simulink model "ECE_431_Homework_6"  (R2017a)
settings: Solver=FixedStepAuto  StartTime=0.0  StopTime=.1  FixedStep=1e-6  MaxStep=1e-4  RelTol=1e-3  EnableMultiTasking=on
undefined symbols (not defined in the file or in its folder): why
libraries: powerlib x9, powerlib_meascontrol x1
settings Model: Creator=Thomas  LastModifiedBy=Kenzie Brian

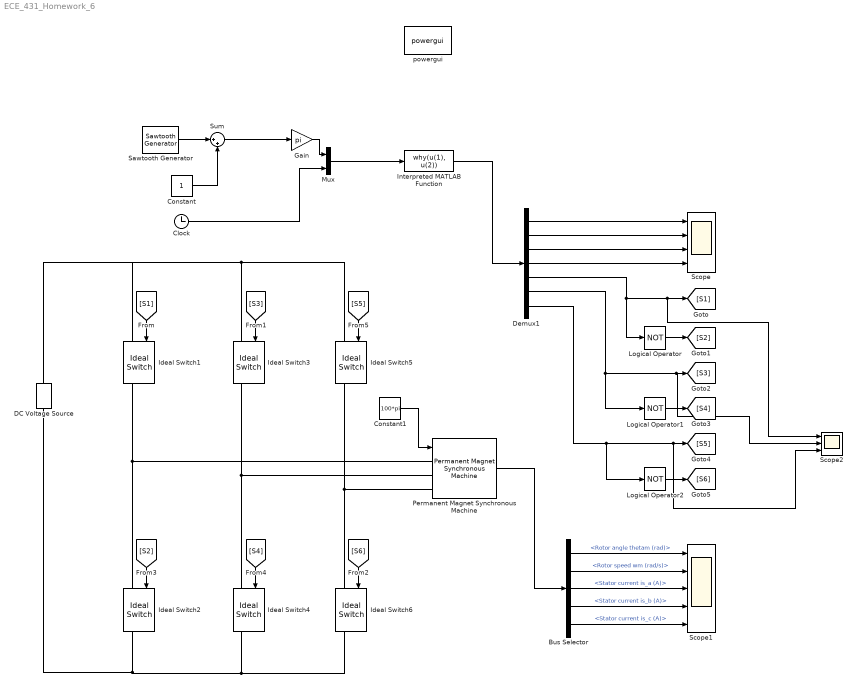
== system ECE_431_Homework_6 ==
  Bus Selector : BusSelector  OutputSignals=Rotor angle thetam (rad),Rotor speed wm (rad/s),Stator current is_a (A),Stator current is_b (A),Stator current is_c (A)
  Clock : Clock
      settings: Decimation=10000
  Constant : Constant
  Constant1 : Constant  Value=100*pi
  DC Voltage Source : powerlib/Electrical Sources/DC Voltage Source  Amplitude=280  Measurements=None
  Demux1 : Demux  Outputs=7
  Gain : Gain  Gain=pi
  Ideal Switch{1..6} (6 alike) : powerlib/Power Electronics/Ideal Switch  Ron=.01  Lon=0  IC=0  Rs=1e5  Cs=inf  Measurements=on
  Interpreted MATLAB Function : MATLABFcn  MATLABFcn=why(u(1), u(2))  Output1D=off
  Logical Operator : Logic  Operator=NOT  AllPortsSameDT=off  OutDataTypeStr=boolean
  Logical Operator1 : Logic  Operator=NOT  AllPortsSameDT=off  OutDataTypeStr=boolean
  Logical Operator2 : Logic  Operator=NOT  AllPortsSameDT=off  OutDataTypeStr=boolean
  Mux : Mux  Inputs=2
  Permanent Magnet Synchronous Machine : powerlib/Machines/Permanent Magnet Synchronous Machine  NbPhases=3  FluxDistribution=Sinusoidal  RotorType=Round  MechanicalLoad=Speed w  PresetModel=No  ShowDetailedParameters=on  MeasurementBus=off  Resistance=0.02  Inductance=8.5e-3  dqInductances=[8.5e-3,8.5e-3]  La=0.0002  MachineConstant=Flux linkage established by magnets (V.s)  Flux=0.03  VoltageCst=21.7656  TorqueCst=0.18  Flat=120  Mechanical=[0.1 0.003 8 0]  PolePairs=4  InitialConditions=[100*pi,0, 0,0]  InitialConditions5ph=[0 0 0 0 0 0]  TsPowergui=0  TsBlock=-1  RefAngle=90 degrees behind phase A axis (modified Park)
      settings: SourceProductName=Simscape Power Systems
  Sawtooth Generator : powerlib_meascontrol/Pulse & Signal Generators/Sawtooth Generator  Freq=100  Phase=180  Ts=0
      settings: SourceProductName=Simscape Power Systems
  Scope : Scope  NumInputPorts=4
  Scope1 : Scope  NumInputPorts=5
  Scope2 : Scope  NumInputPorts=3
  Sum : Sum  Inputs=|++
  powergui : powerlib/powergui  Priority=1  SimulationMode=Discrete  SampleTime=1e-6  frequency=60  Iterations=50  frequencyindice=0  Pbase=100e6  ErrMax=1e-4  UnitsV=kV  UnitsW=MW  buscounter=0  FunctionMessages=off  echomessages=off  EnableUseOfTLC=off  CurrentSourceSwitches=off  DisableSnubberDevices=off  DisableRonSwitches=off  DisableVfSwitches=off  DisplayEquations=off  SolverType=Tustin/Backward Euler (TBE)  Interpol=off  ExternalGateDelay=off  methode=off  Ts=100  x0status=blocks  SPID=off  SwTol=0  HookPort=off  RestoreLinks=warning  ResistiveCurrentMeasurement=off  Frange=[0:2:500]  Ylog=off  Xlog=on  ShowGrid=off  save=off  variable=ZData  structure=0  ZoomFFT=off  StartTime=0.0  cycles=1  DisplayStyle=1  fundamental=60  FreqAxis=off  MaxFrequency=1000  frequencyindicesteady=1  RmsSteady=1  display=off
  wires:
  Sawtooth Generator/1 -> Sum/1
  Mux/1 -> Interpreted MATLAB Function/1
  Constant/1 -> Sum/2
  Clock/1 -> Mux/2
  Demux1/2 -> Scope/2
  Demux1/3 -> Scope/3
  Sum/1 -> Gain/1
  Demux1/1 -> Scope/1
  Interpreted MATLAB Function/1 -> Demux1/1
  Demux1/4 -> Scope/4
  Gain/1 -> Mux/1
  [S3] -> Ideal Switch3/1
  [S1] -> Ideal Switch1/1
  [S5] -> Ideal Switch5/1
  [S2] -> Ideal Switch2/1
  [S4] -> Ideal Switch4/1
  [S6] -> Ideal Switch6/1
  Logical Operator/1 -> [S2]
  Logical Operator2/1 -> [S6]
  Logical Operator1/1 -> [S4]
  Demux1/6 -> Scope2/2, [S3], Logical Operator1/1
  Demux1/5 -> Scope2/1, [S1], Logical Operator/1
  Demux1/7 -> Scope2/3, [S5], Logical Operator2/1
  Permanent Magnet Synchronous Machine/1 -> Bus Selector/1
  Bus Selector/1 -> Scope1/1  "<Rotor angle thetam (rad)>"
  Bus Selector/2 -> Scope1/2  "<Rotor speed wm (rad/s)>"
  Bus Selector/3 -> Scope1/3  "<Stator current is_a (A)>"
  Bus Selector/4 -> Scope1/4  "<Stator current is_b (A)>"
  Bus Selector/5 -> Scope1/5  "<Stator current is_c (A)>"
  Constant1/1 -> Permanent Magnet Synchronous Machine/1
  connections:
  Ideal Switch2/LConn1 -- Permanent Magnet Synchronous Machine/LConn1 -- Ideal Switch1/RConn1
  Ideal Switch3/RConn1 -- Permanent Magnet Synchronous Machine/LConn2 -- Ideal Switch4/LConn1
  Ideal Switch6/LConn1 -- Permanent Magnet Synchronous Machine/LConn3 -- Ideal Switch5/RConn1
  Ideal Switch5/LConn1 -- DC Voltage Source/RConn1 -- Ideal Switch1/LConn1 -- Ideal Switch3/LConn1
  Ideal Switch2/RConn1 -- DC Voltage Source/LConn1 -- Ideal Switch6/RConn1 -- Ideal Switch4/RConn1
